simulink model "car"  (R2018a)
settings: Solver=VariableStepAuto  StartTime=tmin  StopTime=tmax  RelTol=1e-3
values from neighbouring files (symbols this model uses):
  d = 1    [L13T2.m]
  f0 = [ 1 2 deg2rad(45) deg2rad(0) deg2rad(0) ]    [L13T2.m]
  l = 2    [L13T2.m]
settings Model: Creator=meron  LastModifiedBy=meron

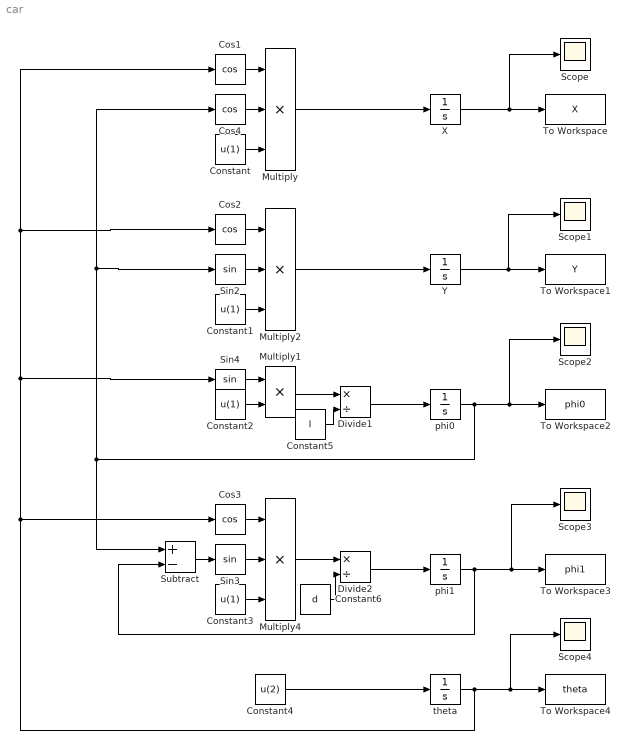
== system car ==
  Constant{,1..3} (4 alike) : Constant  Value=u(1)
  Constant4 : Constant  Value=u(2)
  Constant5 : Constant  Value=l
  Constant6 : Constant  Value=d
  Cos{1..4} (4 alike) : Trigonometry  Operator=cos
  Divide1 : Product  Inputs=*/
  Divide2 : Product  Inputs=*/
  Multiply : Product  Inputs=3
  Multiply1 : Product
  Multiply2 : Product  Inputs=3
  Multiply4 : Product  Inputs=3
  Scope{,1..4} (5 alike) : Scope
  Sin2 : Trigonometry
  Sin3 : Trigonometry
  Sin4 : Trigonometry
  Subtract : Sum  Inputs=+-
  To Workspace : ToWorkspace  VariableName=X  SampleTime=-1
  To Workspace1 : ToWorkspace  VariableName=Y  SampleTime=-1
  To Workspace2 : ToWorkspace  VariableName=phi0  SampleTime=-1
  To Workspace3 : ToWorkspace  VariableName=phi1  SampleTime=-1
  To Workspace4 : ToWorkspace  VariableName=theta  SampleTime=-1
  X : Integrator  InitialCondition=f0(1)
  Y : Integrator  InitialCondition=f0(2)
  phi0 : Integrator  InitialCondition=f0(4)
  phi1 : Integrator  InitialCondition=f0(3)
  theta : Integrator  InitialCondition=f0(5)
  wires:
  Cos1/1 -> Multiply/1
  Cos2/1 -> Multiply2/1
  Cos4/1 -> Multiply/2
  Sin2/1 -> Multiply2/2
  Constant/1 -> Multiply/3
  Constant1/1 -> Multiply2/3
  Multiply1/1 -> Divide1/1
  Constant4/1 -> theta/1
  Divide1/1 -> phi0/1
  Cos3/1 -> Multiply4/1
  Sin3/1 -> Multiply4/2
  Constant3/1 -> Multiply4/3
  Constant2/1 -> Multiply1/2
  Sin4/1 -> Multiply1/1
  Multiply4/1 -> Divide2/1
  Divide2/1 -> phi1/1
  Multiply2/1 -> Y/1
  Multiply/1 -> X/1
  theta/1 -> Scope4/1, To Workspace4/1, Sin4/1, Cos2/1, Cos1/1, Cos3/1
  phi0/1 -> Scope2/1, To Workspace2/1, Subtract/1, Sin2/1, Cos4/1
  Subtract/1 -> Sin3/1
  phi1/1 -> Scope3/1, To Workspace3/1, Subtract/2
  X/1 -> Scope/1, To Workspace/1
  Y/1 -> Scope1/1, To Workspace1/1
  Constant5/1 -> Divide1/2
  Constant6/1 -> Divide2/2
